simulink model "Model_Verification"  (R2018b)
settings: Solver=VariableStepAuto  StartTime=0.0  StopTime=10  RelTol=1e-3
settings Model: Creator=rtana  LastModifiedBy=rtana

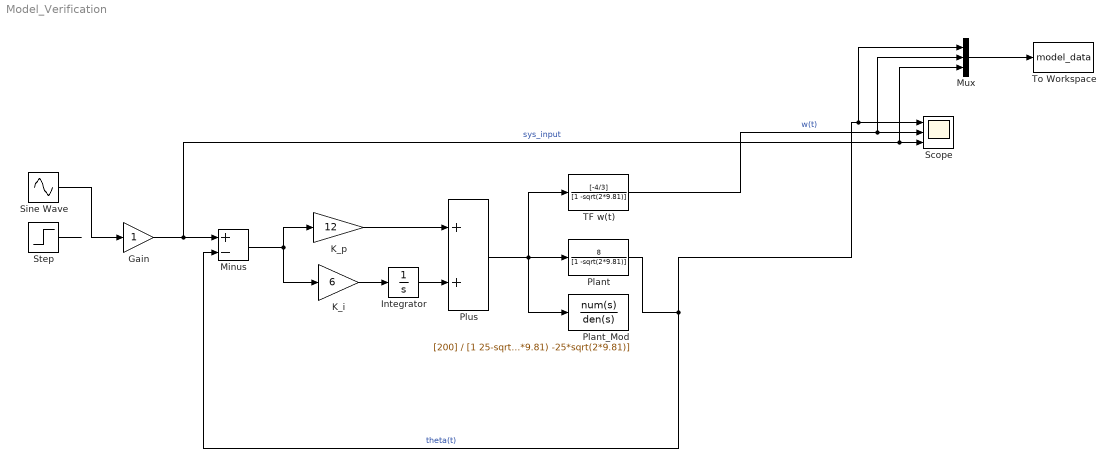
== system Model_Verification ==
  Gain : Gain
  Integrator : Integrator
  K_i : Gain  Gain=6
  K_p : Gain  Gain=12
  Minus : Sum  Inputs=+-
  Mux : Mux  Inputs=3
  Plant : TransferFcn  Numerator=[8]  Denominator=[1 -sqrt(2*9.81)]
  Plant_Mod : TransferFcn  Numerator=[200]  Denominator=[1 25-sqrt(2*9.81) -25*sqrt(2*9.81)]
  Plus : Sum
  Scope : Scope  NumInputPorts=3
  Sine Wave : Sin  Frequency=0.5  SampleTime=0
  Step : Step  After=0.5  SampleTime=0
  TF w(t) : TransferFcn  Numerator=[-4/3]  Denominator=[1 -sqrt(2*9.81)]
  To Workspace : ToWorkspace  VariableName=model_data  SaveFormat=Timeseries  SampleTime=-1
  wires:
  Step/1 -> ?
  K_i/1 -> Integrator/1
  Minus/1 -> K_p/1, K_i/1
  K_p/1 -> Plus/1
  Integrator/1 -> Plus/2
  Plus/1 -> Plant_Mod/1, TF w(t)/1, Plant/1
  TF w(t)/1 -> Mux/2, Scope/2  "w(t)"
  Gain/1 -> Mux/3, Scope/3, Minus/1  "sys_input"
  Plant/1 -> Mux/1, Scope/1, Minus/2  "theta(t)"
  Mux/1 -> To Workspace/1
  Sine Wave/1 -> Gain/1
